simulink model "continous_math_model"  (R2022a)
settings: Solver=FixedStepDiscrete  StartTime=0.0  StopTime=10.0  FixedStep=1  RelTol=1e-3
settings Model: Creator=12191  LastModifiedBy=12191
settings OptimizationCC: DefaultParameterBehavior=Inlined  EnhancedBackFolding=on  PassReuseOutputArgsAs=Individual arguments  ZeroExternalMemoryAtStartup=off  ZeroInternalMemoryAtStartup=off  OptimizeBlockOrder=speed  DifferentSizesBufferReuse=on  OptimizationCustomize=off  EfficientTunableParamExpr=on
settings DebuggingCC: ParameterTunabilityLossMsg=error
settings SFSimCC: MATLABDynamicMemAlloc=off
settings RTWCC: SystemTargetFile=ert.tlc  GenCodeOnly=on  PackageGeneratedCodeAndArtifacts=on  PackageName=calculate  TemplateMakefile=ert_default_tmf  Toolchain=Microsoft Visual C++ 2019 v16.0 | nmake (64-bit Windows)  TargetLang=C++
settings CodeAppCC: ForceParamTrailComments=on  IgnoreCustomStorageClasses=off  OperatorAnnotations=on  SimulinkDataObjDesc=on  SFDataObjDesc=on  InsertBlockDesc=on
settings ERTTargetCC: TargetLangStandard=C++11 (ISO)  GenerateSampleERTMain=on  CodeInterfacePackaging=C++ class  InlinedParameterPlacement=NonHierarchical  RootIOFormat=Structure reference  ERTCustomFileTemplate=example_file_process.tlc

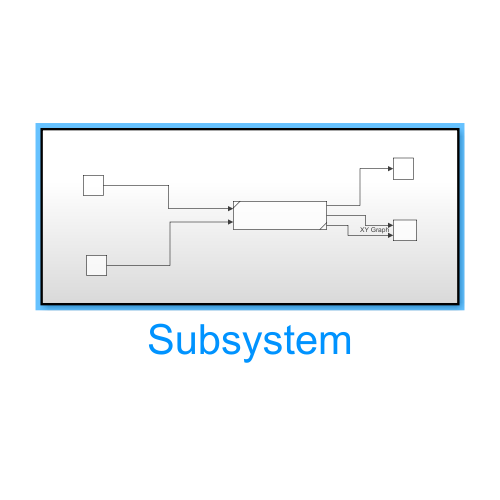
[thumbnail: Simulink's stored preview of the top-level diagram]
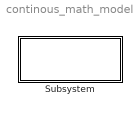
== system continous_math_model ==
  Subsystem : Subsystem

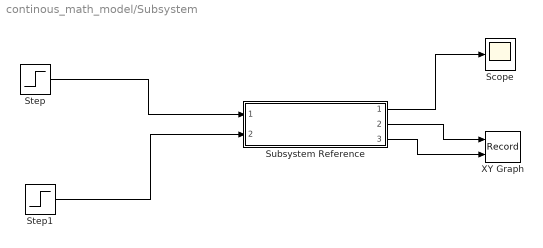
== system continous_math_model/Subsystem ==
  Scope : Scope
  Step : Step  Time=5  After=45  SampleTime=0
  Step1 : Step  Time=0  After=5  SampleTime=0
  Subsystem Reference : Subsystem  ReferencedSubsystem=Drive_d
  XY Graph : Record  FileSettingsInternal="{\"entries\":[{\"content\":{\"excelSettings\":{\"content\":{},\"type\":\"Streamout.ExcelSettings\"}},\"type\":\"Streamout.FileSettingStorage\",\"uuid\":\"2e9b3d65-02e3-49c6-a4b5-29d42d79beb1\"}],\"packageUris\":[\"http://schema.mathworks.com/mf0/streamout_blocks/R2020a\"],\"version\":\"1.0\"}"  Layout=[1 1]  SignalsInternal="{\"entries\":[{\"content\":{\"signals\":[{\"content\":{\"blockPath\":[\"c_ex/Subsystem/XY Graph\"],\"channel\":[],\"dimensions\":[1],\"domain\":\"c_ex/Subsystem/XY Graph\",\"lineColor\":\"#a2142f\",\"plots\":[1],\"port\":1,\"sid\":[],\"signalID\":27,\"signalName\":\"Subsystem Reference:2\"},\"type\":\"RecordBlkView.Signal\",\"uuid\":\"9d218487-7b4f-4588-8455-3128b340ae2c\"},{\"content\":{\"blockPath\":[\"c_ex/Subsystem/XY Graph\"],\"channel\":[],\"dimensions\":[1],\"domain\":\"c_ex/Subsystem/XY Graph\",\"lineColor\":\"#139fff\",\"plots\":[1],\"port\":2,\"sid\":[],\"signalID\":30,\"signalName\":\"Subsystem Reference:3\"},\"type\":\"RecordBlkView.Signal\",\"uuid\":\"8cd63352-d195-451e-b4b6-25a186a74df8\"}]},\"type\":\"RecordBlkView.InputSignals\",\"uuid\":\"9ed10558-3495-4527-b495-04ce8435372c\"}],\"packageUris\":[\"http://schema.mathworks.com/mf0/streamout_blocks/R2020a\"],\"version\":\"1.0\"}"  VisualizationBindings="{\"xyplotplugin\":{\"info\":[{\"series\":[{\"bindingParametersList\":[{\"parameter\":\"X-Axis\",\"signalID\":27,\"signalName\":\"Subsystem Reference:2\"},{\"parameter\":\"Y-Axis\",\"signalID\":30,\"signalName\":\"Subsystem Reference:3\"}],\"seriesID\":5038}],\"subplotID\":1}]}}"  CompatibilityTag=XY
  wires:
  Step/1 -> Subsystem Reference/1
  Step1/1 -> Subsystem Reference/2
  Subsystem Reference/1 -> Scope/1
  Subsystem Reference/2 -> XY Graph/1
  Subsystem Reference/3 -> XY Graph/2
